simulink model "WirkungsplanEuler"  (R2021b)
settings: Solver=ode1  StartTime=0.0  StopTime=10.0  FixedStep=dt  RelTol=1e-3
values from neighbouring files (symbols this model uses):
  a0 = 1    [Euler.m]    (also in Euler_Nur_PT1.m)
  a1 = 1    [Euler.m]
  b0 = 1    [Euler.m]    (also in Euler_Nur_PT1.m)
  b1 = 1    [Euler.m]
  b2 = 0    [Euler.m]
settings Model: Creator=PM  LastModifiedBy=PM

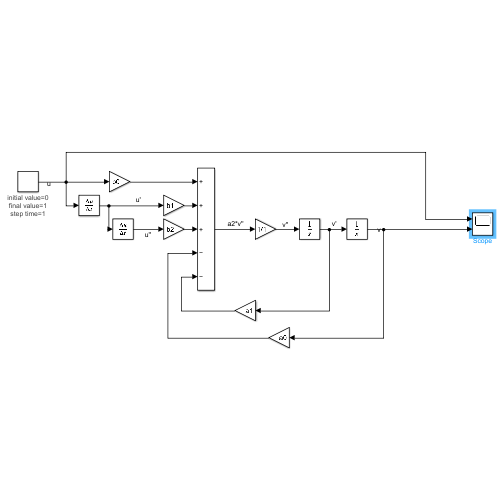
[thumbnail: Simulink's stored preview of the top-level diagram]
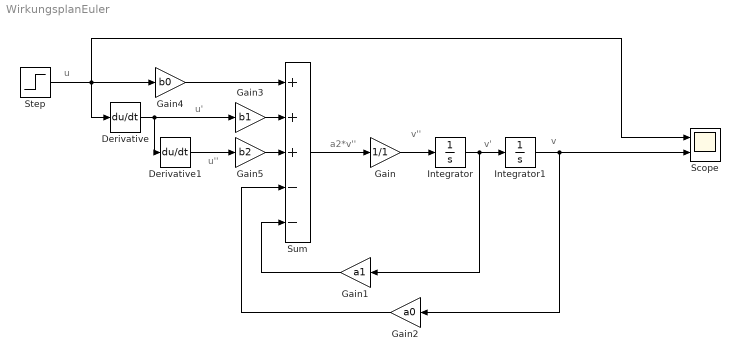
== system WirkungsplanEuler ==
  note: u''
  note: u'
  note: u
  note: v
  note: v'
  note: v''
  note: a2*v''
  Derivative : Derivative
  Derivative1 : Derivative
  Gain : Gain  Gain=1/1
  Gain1 : Gain  Gain=a1
  Gain2 : Gain  Gain=a0
  Gain3 : Gain  Gain=b1
  Gain4 : Gain  Gain=b0
  Gain5 : Gain  Gain=b2
  Integrator : Integrator
  Integrator1 : Integrator
  Scope : Scope  NumInputPorts=2
  Step : Step  SampleTime=0
      settings: AttributesFormatString=initial value=%<Before>\nfinal value=%<After>\nstep time=%<Time>
  Sum : Sum  Inputs=+++--
  wires:
  Sum/1 -> Gain/1
  Gain/1 -> Integrator/1
  Integrator/1 -> Gain1/1, Integrator1/1
  Integrator1/1 -> Gain2/1, Scope/2
  Gain1/1 -> Sum/5
  Gain2/1 -> Sum/4
  Derivative/1 -> Derivative1/1, Gain3/1
  Gain3/1 -> Sum/2
  Gain4/1 -> Sum/1
  Gain5/1 -> Sum/3
  Derivative1/1 -> Gain5/1
  Step/1 -> Scope/1, Derivative/1, Gain4/1
